simulink model "CF010A_GmTqArbn"  (R2013b)
settings: Solver=FixedStepDiscrete  SolverMode=SingleTasking  StartTime=0.0  StopTime=1  FixedStep=0.002  RelTol=1e-3
values from neighbouring files (symbols this model uses):
  ARCHGLBPRM_2MILLISEC_SEC_F32 = DataDict.Constant    [CF010A_GmTqArbn_DataDict.m]
  ESCTQCMDOVRLLIM_HWNWTMTR_F32 = DataDict.Constant    [CF010A_GmTqArbn_DataDict.m]
  FINALSLEWLWRLIM_HWNWTMTRPERSEC_F32 = DataDict.Constant    [CF010A_GmTqArbn_DataDict.m]
  GmTqArbnApaAssiScaEna = DataDict.Calibration    [CF010A_GmTqArbn_DataDict.m]
  GmTqArbnApaDampgScaEna = DataDict.Calibration    [CF010A_GmTqArbn_DataDict.m]
  GmTqArbnApaEnaRate = DataDict.Calibration    [CF010A_GmTqArbn_DataDict.m]
  GmTqArbnApaRtnScaEna = DataDict.Calibration    [CF010A_GmTqArbn_DataDict.m]
  GmTqArbnEscMaxTq = DataDict.Calibration    [CF010A_GmTqArbn_DataDict.m]
  GmTqArbnLkaOutpOvrlUpprLim = DataDict.Calibration    [CF010A_GmTqArbn_DataDict.m]
  GmTqArbnLkaSlewEna = DataDict.Calibration    [CF010A_GmTqArbn_DataDict.m]
  HWTQCMDOVRLLIM_HWNWTMTR_F32 = DataDict.Constant    [CF010A_GmTqArbn_DataDict.m]
  LKACMDHILIM_HWNWTMTR_F32 = DataDict.Constant    [CF010A_GmTqArbn_DataDict.m]
  LKAOUTPOVRLLIM_MOTNWTMTR_F32 = DataDict.Constant    [CF010A_GmTqArbn_DataDict.m]
  LKATQCMDOVRLLIM_HWNWTMTR_F32 = DataDict.Constant    [CF010A_GmTqArbn_DataDict.m]
  MOTTQCMDOVRLLIM_MOTNWTMTR_F32 = DataDict.Constant    [CF010A_GmTqArbn_DataDict.m]
  OUTPCMDHILIM_ULS_F32 = DataDict.Constant    [CF010A_GmTqArbn_DataDict.m]
  OUTPCMDLOWRLIM_ULS_F32 = DataDict.Constant    [CF010A_GmTqArbn_DataDict.m]
  POSNSERVOSMOOTHMINLWRLIM_ULSPERSEC_F32 = DataDict.Constant    [CF010A_GmTqArbn_DataDict.m]
  VELDPTTQOVRLMTRCOFFS_HWNWTMTRPERSEC_F32 = DataDict.Constant    [CF010A_GmTqArbn_DataDict.m]
  VELDPTTQOVRLMTRCTQPERVEHSPD_HWNWTMTRPERSECPERKPH_F32 = DataDict.Constant    [CF010A_GmTqArbn_DataDict.m]
undefined symbols (not defined in the file or in its folder): GmTqArbnEscSt1, GmTqArbnLkaSt1
libraries: NxtrLim x12, simulink x10, NexteerUtilities x8, FixdToFloat x4, NxtrAbslt x3, Fil x2, FloatToFixd x2, BilnrIntrpnMplX x1, NxtrSign x1
(part 4 of 5)

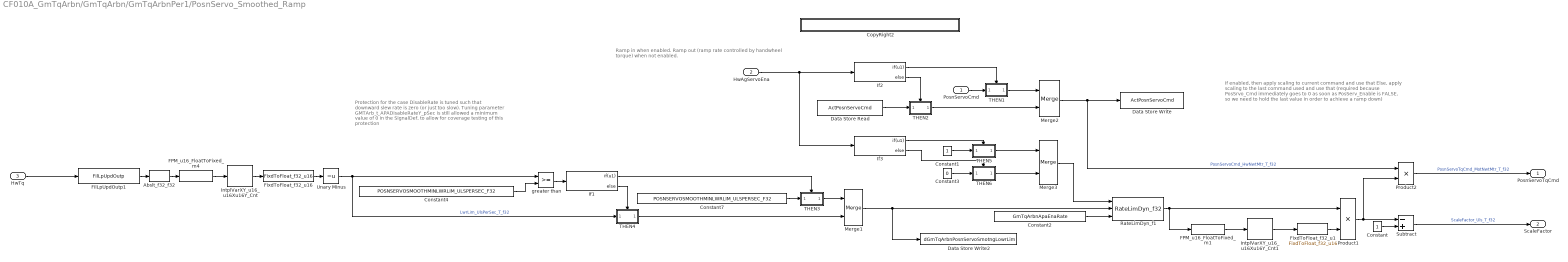
== system CF010A_GmTqArbn/GmTqArbn/GmTqArbnPer1/PosnServo_Smoothed_Ramp ==
  note: Protection for the case DisableRate is tuned such that
      | downward slew rate is zero (or just too slow).
      |
      | Tuning parameter GMTArb_t_APADisableRateY_pSec is still
      | allowed a minimum value of 0 in the SignalDef, to allow for
      | coverage testing of this protection
  note: Ramp in when enabled.
      | Ramp out (ramp rate controlled by handwheel torque) when not enabled.
  note: If enabled,
      |     then apply scaling to current command and use that
      | Else,
      |     apply scaling to the last command used and use that
      |
      |           (required because PosSrvo_Cmd immediately goes to 0 as soon
      |            as PosServ_Enable is FALSE, so we need to hold the last value
      |            in order to achieve a ramp down)
  PosnServoCmd : Inport  RequirementInfo="{'linktype_rmi_doors' '0000c6e3 (/E-STEER Core/SubSystem Specifications/Customer Functions - EA4/GM/CF010A GM Torque Arbitrator)' '#CF010A_83' 'true' 'REQ:  CF010A_83' '' } %GIDa_a589d5a5_5fe7_4259_9e30_a8e3d0a14d84"
  HwAgServoEna : Inport  RequirementInfo="{'linktype_rmi_doors' '0000c6e3 (/E-STEER Core/SubSystem Specifications/Customer Functions - EA4/GM/CF010A GM Torque Arbitrator)' '#CF010A_83' 'true' 'REQ:  CF010A_83' '' } %GIDa_3c39fabe_76d8_4d75_b934_ff4ece5048a2"  Port=2
  HwTq : Inport  RequirementInfo="{'linktype_rmi_doors' '0000c6e3 (/E-STEER Core/SubSystem Specifications/Customer Functions - EA4/GM/CF010A GM Torque Arbitrator)' '#CF010A_85' 'true' 'REQ:  CF010A_85' '' } %GIDa_14a06130_4ede_469d_aba7_55d801ee6fbb"  Port=3
  Abslt_f32_f32 : NxtrAbslt/Abslt_f32_f32  RequirementInfo="{'linktype_rmi_doors' '0000c6e3 (/E-STEER Core/SubSystem Specifications/Customer Functions - EA4/GM/CF010A GM Torque Arbitrator)' '#CF010A_85' 'true' 'REQ:  CF010A_85' '' } %GIDa_1d732af2_bae1_4918_9fbb_75956b3de41a"  SFunctionSpec=single y1 = Abslt_f32_f32(single u1)
      settings: AttributesFormatString=%<Name>
  Constant : Constant  RequirementInfo="{'linktype_rmi_doors' '0000c6e3 (/E-STEER Core/SubSystem Specifications/Customer Functions - EA4/GM/CF010A GM Torque Arbitrator)' '#CF010A_87' 'true' 'REQ:  CF010A_87' '' } %GIDa_6652223e_5f9e_4f22_b2f7_82ef07e16371"  OutDataTypeStr=single
  Constant1 : Constant  RequirementInfo="{'linktype_rmi_doors' '0000c6e3 (/E-STEER Core/SubSystem Specifications/Customer Functions - EA4/GM/CF010A GM Torque Arbitrator)' '#CF010A_83' 'true' 'REQ:  CF010A_83' '' } %GIDa_8a974f93_c71b_4ff7_97b8_e3459b4cb0d6"  OutDataTypeStr=single
  Constant2 : Constant  RequirementInfo="{'linktype_rmi_doors' '0000c6e3 (/E-STEER Core/SubSystem Specifications/Customer Functions - EA4/GM/CF010A GM Torque Arbitrator)' '#CF010A_84' 'true' 'REQ:  CF010A_84' '' } %GIDa_7ed8c832_ce99_4127_9a80_eb8922502510"  Value=GmTqArbnApaEnaRate
  Constant3 : Constant  RequirementInfo="{'linktype_rmi_doors' '0000c6e3 (/E-STEER Core/SubSystem Specifications/Customer Functions - EA4/GM/CF010A GM Torque Arbitrator)' '#CF010A_83' 'true' 'REQ:  CF010A_83' '' } %GIDa_389fbbe5_3959_44b2_9e53_45f6397d449f"  Value=0  OutDataTypeStr=single
  Constant4 : Constant  RequirementInfo={} %GIDa_c73b5d52_2f1d_4595_892c_5347f865968c  Value=POSNSERVOSMOOTHMINLWRLIM_ULSPERSEC_F32
  Constant7 : Constant  RequirementInfo={} %GIDa_8f1476cf_19b2_4cf1_8322_e9f8d22341c9  Value=POSNSERVOSMOOTHMINLWRLIM_ULSPERSEC_F32
  CopyRight2 : Subsystem  Description=|  mask(Copyright Information){none=on}
      | Copyright info block.                                               
      |                                                                     
      | Place copyright information at the top of every subsystem in design.
      mask prompts: none "No parameters"
      mask help: Place copyright information at the top of every subsystem in design.
      mask Display:
      | NxtrConf = 'Nexteer Confidential';
      | 
      | sys = bdroot; %handle for the current model ("system")
      | first = get_param(sys,'Created');
      | first = first(end-3:end);  %year is last four digits
      | 
      | last = get_param(sys,'LastModifiedDate');
      | if isempty(last)
      |     last = datestr(now,'yyyy');
      | else
      |     last = last(end-3:end);
      | end
      | 
      | if strcmp(first,last)
      |     fprintf('%s -- Copyright %s Nexteer',NxtrConf,first)
      | else
      |     fprintf('%s -- %s%s- %s Nexteer',NxtrConf,char(169),first,last)
      | end
  Data Store Read : DataStoreRead  RequirementInfo="{'linktype_rmi_doors' '0000c6e3 (/E-STEER Core/SubSystem Specifications/Customer Functions - EA4/GM/CF010A GM Torque Arbitrator)' '#CF010A_83' 'true' 'REQ:  CF010A_83' '' } %GIDa_2b8eed64_a4c6_49b0_96b2_799e9470223f"  DataStoreName=ActPosnServoCmd
  Data Store Write : DataStoreWrite  RequirementInfo="{'linktype_rmi_doors' '0000c6e3 (/E-STEER Core/SubSystem Specifications/Customer Functions - EA4/GM/CF010A GM Torque Arbitrator)' '#CF010A_83' 'true' 'REQ:  CF010A_83' '' } %GIDa_49e27e17_eee5_40eb_b093_ed4163babafd"  DataStoreName=ActPosnServoCmd
  Data Store Write2 : DataStoreWrite  DataStoreName=dGmTqArbnPosnServoSmotngLowrLim
  FPM_u16_FloatToFixed_m1 : NexteerUtilities/Fixed Point Math Conversions/FPM_u16_FloatToFixed_m  RequirementInfo="{'linktype_rmi_doors' '0000c6e3 (/E-STEER Core/SubSystem Specifications/Customer Functions - EA4/GM/CF010A GM Torque Arbitrator)' '#CF010A_87' 'true' 'REQ:  CF010A_87' '' } %GIDa_42565968_b0f1_480f_9ffe_acf6ef03b720"  SFunctionSpec=uint16 y1 = FPM_u16_FloatToFixed_m(single u1, single p1)  Param1=15
      settings: AttributesFormatString=u16_FloatToFixed
  FPM_u16_FloatToFixed_m4 : NexteerUtilities/Fixed Point Math Conversions/FPM_u16_FloatToFixed_m  RequirementInfo="{'linktype_rmi_doors' '0000c6e3 (/E-STEER Core/SubSystem Specifications/Customer Functions - EA4/GM/CF010A GM Torque Arbitrator)' '#CF010A_85' 'true' 'REQ:  CF010A_85' '' } %GIDa_11a7f01b_449d_4110_953e_6440d8c88ec2"  SFunctionSpec=uint16 y1 = FPM_u16_FloatToFixed_m(single u1, single p1)  Param1=12
      settings: AttributesFormatString=u16_FloatToFixed
  FilLpUpdOutp1 : Fil/FilLpUpdOutp  RequirementInfo="{'linktype_rmi_doors' '0000c6e3 (/E-STEER Core/SubSystem Specifications/Customer Functions - EA4/GM/CF010A GM Torque Arbitrator)' '#CF010A_85' 'true' 'REQ:  CF010A_85' '' } %GIDa_6001f4fc_91a0_455a_8ef8_6b05b3874b38"  StVar=ApaSmotngHwTqLpFil
      settings: AttributesFormatString=StVar: %<StVar>
  FixdToFloat_f32_u1 : FixdToFloat/FixdToFloat_f32_u16  RequirementInfo="{'linktype_rmi_doors' '0000c6e3 (/E-STEER Core/SubSystem Specifications/Customer Functions - EA4/GM/CF010A GM Torque Arbitrator)' '#CF010A_87' 'true' 'REQ:  CF010A_87' '' } %GIDa_01cc822d_a521_45f2_8614_de07a41cf4e7"  Param1=15
  FixdToFloat_f32_u16 : FixdToFloat/FixdToFloat_f32_u16  RequirementInfo="{'linktype_rmi_doors' '0000c6e3 (/E-STEER Core/SubSystem Specifications/Customer Functions - EA4/GM/CF010A GM Torque Arbitrator)' '#CF010A_85' 'true' 'REQ:  CF010A_85' '' } %GIDa_d247bf31_8ee9_41f8_b2ef_9ed7cd29173a"  Param1=9
  If1 : If  RequirementInfo={} %GIDa_446387ce_f822_476d_a5ec_ea0813341457  IfExpression=u1
  If2 : If  RequirementInfo="{'linktype_rmi_doors' '0000c6e3 (/E-STEER Core/SubSystem Specifications/Customer Functions - EA4/GM/CF010A GM Torque Arbitrator)' '#CF010A_83' 'true' 'REQ:  CF010A_83' '' } %GIDa_caed38e4_3d6b_4104_9897_516a2005e0ea"  IfExpression=u1
  If3 : If  RequirementInfo="{'linktype_rmi_doors' '0000c6e3 (/E-STEER Core/SubSystem Specifications/Customer Functions - EA4/GM/CF010A GM Torque Arbitrator)' '#CF010A_83' 'true' 'REQ:  CF010A_83' '' } %GIDa_cb067983_f98e_478f_9a9b_9a4768f0638b"  IfExpression=u1
  IntplVarXY_u16_u16Xu16Y_Cnt : NexteerUtilities/Interpolation/IntplVarXY_u16_u16Xu16Y_Cnt  RequirementInfo="{'linktype_rmi_doors' '0000c6e3 (/E-STEER Core/SubSystem Specifications/Customer Functions - EA4/GM/CF010A GM Torque Arbitrator)' '#CF010A_85' 'true' 'REQ:  CF010A_85' '' } %GIDa_c034638a_826b_4a44_a2db_ef50f5019c4a"  Param1=GmTqArbnApaDiRateX  Param2=GmTqArbnApaDiRateY
      settings: AttributesFormatString=IntplVarXY (uX, uY)
  IntplVarXY_u16_u16Xu16Y_Cnt1 : NexteerUtilities/Interpolation/IntplVarXY_u16_u16Xu16Y_Cnt  RequirementInfo="{'linktype_rmi_doors' '0000c6e3 (/E-STEER Core/SubSystem Specifications/Customer Functions - EA4/GM/CF010A GM Torque Arbitrator)' '#CF010A_87' 'true' 'REQ:  CF010A_87' '' ; 'linktype_rmi_doors' '0000c6e3 (/E-STEER Core/SubSystem Specifications/Customer Functions - EA4/GM/CF010A GM Torque Arbitrator)' '#CF010A_86' 'true' 'REQ:  CF010A_86' '' } %GIDa_d2f04c6c_cd0d_4f5b_a0ee_624f7a3ac7bb"  Param1=GmTqArbnApaSmotngX  Param2=GmTqArbnApaSmotngY
      settings: AttributesFormatString=IntplVarXY (uX, uY)
  Merge1 : Merge  RequirementInfo={} %GIDa_c6bad38d_cfbe_4ba5_8efa_e31f6e6c40e4
  Merge2 : Merge  RequirementInfo="{'linktype_rmi_doors' '0000c6e3 (/E-STEER Core/SubSystem Specifications/Customer Functions - EA4/GM/CF010A GM Torque Arbitrator)' '#CF010A_83' 'true' 'REQ:  CF010A_83' '' } %GIDa_315cc2c9_a434_4900_996a_ec94b76d111f"
  Merge3 : Merge  RequirementInfo="{'linktype_rmi_doors' '0000c6e3 (/E-STEER Core/SubSystem Specifications/Customer Functions - EA4/GM/CF010A GM Torque Arbitrator)' '#CF010A_83' 'true' 'REQ:  CF010A_83' '' } %GIDa_22e32ead_0ffe_4af6_9c30_1dceeecbc313"
  Product1 : Product  RequirementInfo="{'linktype_rmi_doors' '0000c6e3 (/E-STEER Core/SubSystem Specifications/Customer Functions - EA4/GM/CF010A GM Torque Arbitrator)' '#CF010A_87' 'true' 'REQ:  CF010A_87' '' } %GIDa_d490a3f1_7ea3_496c_9645_bccc177abc5b"  OutDataTypeStr=single  RndMeth=Zero
  Product2 : Product  RequirementInfo="{'linktype_rmi_doors' '0000c6e3 (/E-STEER Core/SubSystem Specifications/Customer Functions - EA4/GM/CF010A GM Torque Arbitrator)' '#CF010A_86' 'true' 'REQ:  CF010A_86' '' } %GIDa_1ff153b9_865b_4418_aa1c_8853e303e2f0"  OutDataTypeStr=single  RndMeth=Zero
  RateLimDyn_f1 : NxtrLim/RateLimDyn_f32  RequirementInfo="{'linktype_rmi_doors' '0000c6e3 (/E-STEER Core/SubSystem Specifications/Customer Functions - EA4/GM/CF010A GM Torque Arbitrator)' '#CF010A_84' 'true' 'REQ:  CF010A_84' '' } %GIDa_4a1a811f_29b7_4717_8310_006cae323995"  StVar=PosnServoSmotngEnaRateLim  Ts=ARCHGLBPRM_2MILLISEC_SEC_F32
      settings: AttributesFormatString=StVar: %<StVar>
  Subtract : Sum  RequirementInfo="{'linktype_rmi_doors' '0000c6e3 (/E-STEER Core/SubSystem Specifications/Customer Functions - EA4/GM/CF010A GM Torque Arbitrator)' '#CF010A_87' 'true' 'REQ:  CF010A_87' '' } %GIDa_3c2bba99_87d7_4ba6_923a_93c919a35035"  Inputs=-+
  THEN1 : Subsystem  RequirementInfo="{'linktype_rmi_doors' '0000c6e3 (/E-STEER Core/SubSystem Specifications/Customer Functions - EA4/GM/CF010A GM Torque Arbitrator)' '#CF010A_83' 'true' 'REQ:  CF010A_83' '' } %GIDa_80c3f70f_6981_41a7_879d_713cfb9f3918"  TreatAsAtomicUnit=on  mask(pass thru, version Nov 30, 2012){nIn=1}
      mask prompts: nIn "Number of input signals"
      mask help:
      | This block passes its input straight through without modification.
      |
      | Enter the number of signals to pass through (integer 1 to 5).
      mask Callback nIn:
      | thisBlock = gcb;
      | a = get_param(thisBlock,'MaskValues');
      | b = cell2mat(a);
      | c = str2num(b);
      | 
      | if c<1 c=1; end
      | if c>5 c=5; end
      | 
      | for idx=1:c
      |     sIdx = num2str(idx);
      |     oldblock = [thisBlock '/In' sIdx];
      |     if strcmp(get_param(oldblock,'BlockType'),'Ground')
      |          newblock = 'built-in/Inport';
      |         pos = get_param(oldblock,'Position');
      |         orient = get_param(oldblock,'Orientation');
      |         delete_block(oldblock);
      |         add_block(newblock,oldblock,'Position',pos, 'Orientation',orient);
      |     end
      | 
      |     oldblock = [thisBlock '/Out' sIdx];
      |     if strcmp(get_param(oldblock,'BlockType'),'Terminator')
      |         newblock = 'built-in/Outport';
      |         pos = get_param(oldblock,'Position');
      |         orient = get_param(oldblock,'Orientation');
      |         delete_block(oldblock);
      |         add_block(newblock,oldblock,'Position',pos, 'Orientation',orient);
      |     end
      | end
      | 
      | for idx=c+1:5
      |     sIdx = num2str(idx);
      |     oldblock = [thisBlock '/In' sIdx];
      |     if strcmp(get_param(oldblock,'BlockType'),'Inport')
      |         newblock = 'built-in/Ground';
      |         pos = get_param(oldblock,'Position');
      |         orient = get_param(oldblock,'Orientation');
      |         delete_block(oldblock);
      |         add_block(newblock,oldblock,'Position',pos, 'Orientation',orient);
      |     end
      | 
      |     oldblock = [thisBlock '/Out' sIdx];
      |     if strcmp(get_param(oldblock,'BlockType'),'Outport')
      |         newblock = 'built-in/Terminator';
      |         pos = get_param(oldblock,'Position');
      |         orient = get_param(oldblock,'Orientation');
      |         delete_block(oldblock);
      |         add_block(newblock,oldblock,'Position',pos, 'Orientation',orient);
      |     end
      | end
      | 
      | 
      | 
      | clear thisBlock oldblock newblock orient pos a b c idx sIdx ;
      mask Display: fprintf('pass\nthru')
  THEN2 : Subsystem  RequirementInfo="{'linktype_rmi_doors' '0000c6e3 (/E-STEER Core/SubSystem Specifications/Customer Functions - EA4/GM/CF010A GM Torque Arbitrator)' '#CF010A_83' 'true' 'REQ:  CF010A_83' '' } %GIDa_f9d28e7a_0d49_44fe_8c5c_4cae6e915892"  TreatAsAtomicUnit=on  mask(pass thru, version Nov 30, 2012){nIn=1}
      mask prompts: nIn "Number of input signals"
      mask help:
      | This block passes its input straight through without modification.
      |
      | Enter the number of signals to pass through (integer 1 to 5).
      mask Callback nIn:
      | thisBlock = gcb;
      | a = get_param(thisBlock,'MaskValues');
      | b = cell2mat(a);
      | c = str2num(b);
      | 
      | if c<1 c=1; end
      | if c>5 c=5; end
      | 
      | for idx=1:c
      |     sIdx = num2str(idx);
      |     oldblock = [thisBlock '/In' sIdx];
      |     if strcmp(get_param(oldblock,'BlockType'),'Ground')
      |          newblock = 'built-in/Inport';
      |         pos = get_param(oldblock,'Position');
      |         orient = get_param(oldblock,'Orientation');
      |         delete_block(oldblock);
      |         add_block(newblock,oldblock,'Position',pos, 'Orientation',orient);
      |     end
      | 
      |     oldblock = [thisBlock '/Out' sIdx];
      |     if strcmp(get_param(oldblock,'BlockType'),'Terminator')
      |         newblock = 'built-in/Outport';
      |         pos = get_param(oldblock,'Position');
      |         orient = get_param(oldblock,'Orientation');
      |         delete_block(oldblock);
      |         add_block(newblock,oldblock,'Position',pos, 'Orientation',orient);
      |     end
      | end
      | 
      | for idx=c+1:5
      |     sIdx = num2str(idx);
      |     oldblock = [thisBlock '/In' sIdx];
      |     if strcmp(get_param(oldblock,'BlockType'),'Inport')
      |         newblock = 'built-in/Ground';
      |         pos = get_param(oldblock,'Position');
      |         orient = get_param(oldblock,'Orientation');
      |         delete_block(oldblock);
      |         add_block(newblock,oldblock,'Position',pos, 'Orientation',orient);
      |     end
      | 
      |     oldblock = [thisBlock '/Out' sIdx];
      |     if strcmp(get_param(oldblock,'BlockType'),'Outport')
      |         newblock = 'built-in/Terminator';
      |         pos = get_param(oldblock,'Position');
      |         orient = get_param(oldblock,'Orientation');
      |         delete_block(oldblock);
      |         add_block(newblock,oldblock,'Position',pos, 'Orientation',orient);
      |     end
      | end
      | 
      | 
      | 
      | clear thisBlock oldblock newblock orient pos a b c idx sIdx ;
      mask Display: fprintf('pass\nthru')
  THEN3 : Subsystem  RequirementInfo={} %GIDa_d57778e5_423b_47fa_b317_4be07015d79c  TreatAsAtomicUnit=on  mask(pass thru, version Nov 30, 2012){nIn=1}
      mask prompts: nIn "Number of input signals"
      mask help:
      | This block passes its input straight through without modification.
      |
      | Enter the number of signals to pass through (integer 1 to 5).
      mask Callback nIn:
      | thisBlock = gcb;
      | a = get_param(thisBlock,'MaskValues');
      | b = cell2mat(a);
      | c = str2num(b);
      | 
      | if c<1 c=1; end
      | if c>5 c=5; end
      | 
      | for idx=1:c
      |     sIdx = num2str(idx);
      |     oldblock = [thisBlock '/In' sIdx];
      |     if strcmp(get_param(oldblock,'BlockType'),'Ground')
      |          newblock = 'built-in/Inport';
      |         pos = get_param(oldblock,'Position');
      |         orient = get_param(oldblock,'Orientation');
      |         delete_block(oldblock);
      |         add_block(newblock,oldblock,'Position',pos, 'Orientation',orient);
      |     end
      | 
      |     oldblock = [thisBlock '/Out' sIdx];
      |     if strcmp(get_param(oldblock,'BlockType'),'Terminator')
      |         newblock = 'built-in/Outport';
      |         pos = get_param(oldblock,'Position');
      |         orient = get_param(oldblock,'Orientation');
      |         delete_block(oldblock);
      |         add_block(newblock,oldblock,'Position',pos, 'Orientation',orient);
      |     end
      | end
      | 
      | for idx=c+1:5
      |     sIdx = num2str(idx);
      |     oldblock = [thisBlock '/In' sIdx];
      |     if strcmp(get_param(oldblock,'BlockType'),'Inport')
      |         newblock = 'built-in/Ground';
      |         pos = get_param(oldblock,'Position');
      |         orient = get_param(oldblock,'Orientation');
      |         delete_block(oldblock);
      |         add_block(newblock,oldblock,'Position',pos, 'Orientation',orient);
      |     end
      | 
      |     oldblock = [thisBlock '/Out' sIdx];
      |     if strcmp(get_param(oldblock,'BlockType'),'Outport')
      |         newblock = 'built-in/Terminator';
      |         pos = get_param(oldblock,'Position');
      |         orient = get_param(oldblock,'Orientation');
      |         delete_block(oldblock);
      |         add_block(newblock,oldblock,'Position',pos, 'Orientation',orient);
      |     end
      | end
      | 
      | 
      | 
      | clear thisBlock oldblock newblock orient pos a b c idx sIdx ;
      mask Display: fprintf('pass\nthru')
  THEN4 : Subsystem  RequirementInfo={} %GIDa_3f4dfbb6_d451_4e7e_94d4_863f405e7908  TreatAsAtomicUnit=on  mask(pass thru, version Nov 30, 2012){nIn=1}
      mask prompts: nIn "Number of input signals"
      mask help:
      | This block passes its input straight through without modification.
      |
      | Enter the number of signals to pass through (integer 1 to 5).
      mask Callback nIn:
      | thisBlock = gcb;
      | a = get_param(thisBlock,'MaskValues');
      | b = cell2mat(a);
      | c = str2num(b);
      | 
      | if c<1 c=1; end
      | if c>5 c=5; end
      | 
      | for idx=1:c
      |     sIdx = num2str(idx);
      |     oldblock = [thisBlock '/In' sIdx];
      |     if strcmp(get_param(oldblock,'BlockType'),'Ground')
      |          newblock = 'built-in/Inport';
      |         pos = get_param(oldblock,'Position');
      |         orient = get_param(oldblock,'Orientation');
      |         delete_block(oldblock);
      |         add_block(newblock,oldblock,'Position',pos, 'Orientation',orient);
      |     end
      | 
      |     oldblock = [thisBlock '/Out' sIdx];
      |     if strcmp(get_param(oldblock,'BlockType'),'Terminator')
      |         newblock = 'built-in/Outport';
      |         pos = get_param(oldblock,'Position');
      |         orient = get_param(oldblock,'Orientation');
      |         delete_block(oldblock);
      |         add_block(newblock,oldblock,'Position',pos, 'Orientation',orient);
      |     end
      | end
      | 
      | for idx=c+1:5
      |     sIdx = num2str(idx);
      |     oldblock = [thisBlock '/In' sIdx];
      |     if strcmp(get_param(oldblock,'BlockType'),'Inport')
      |         newblock = 'built-in/Ground';
      |         pos = get_param(oldblock,'Position');
      |         orient = get_param(oldblock,'Orientation');
      |         delete_block(oldblock);
      |         add_block(newblock,oldblock,'Position',pos, 'Orientation',orient);
      |     end
      | 
      |     oldblock = [thisBlock '/Out' sIdx];
      |     if strcmp(get_param(oldblock,'BlockType'),'Outport')
      |         newblock = 'built-in/Terminator';
      |         pos = get_param(oldblock,'Position');
      |         orient = get_param(oldblock,'Orientation');
      |         delete_block(oldblock);
      |         add_block(newblock,oldblock,'Position',pos, 'Orientation',orient);
      |     end
      | end
      | 
      | 
      | 
      | clear thisBlock oldblock newblock orient pos a b c idx sIdx ;
      mask Display: fprintf('pass\nthru')
  THEN5 : Subsystem  RequirementInfo="{'linktype_rmi_doors' '0000c6e3 (/E-STEER Core/SubSystem Specifications/Customer Functions - EA4/GM/CF010A GM Torque Arbitrator)' '#CF010A_83' 'true' 'REQ:  CF010A_83' '' } %GIDa_1fd1b70b_60eb_42bd_bdff_5612c0d9123a"  TreatAsAtomicUnit=on  mask(pass thru, version Nov 30, 2012){nIn=1}
      mask prompts: nIn "Number of input signals"
      mask help:
      | This block passes its input straight through without modification.
      |
      | Enter the number of signals to pass through (integer 1 to 5).
      mask Callback nIn:
      | thisBlock = gcb;
      | a = get_param(thisBlock,'MaskValues');
      | b = cell2mat(a);
      | c = str2num(b);
      | 
      | if c<1 c=1; end
      | if c>5 c=5; end
      | 
      | for idx=1:c
      |     sIdx = num2str(idx);
      |     oldblock = [thisBlock '/In' sIdx];
      |     if strcmp(get_param(oldblock,'BlockType'),'Ground')
      |          newblock = 'built-in/Inport';
      |         pos = get_param(oldblock,'Position');
      |         orient = get_param(oldblock,'Orientation');
      |         delete_block(oldblock);
      |         add_block(newblock,oldblock,'Position',pos, 'Orientation',orient);
      |     end
      | 
      |     oldblock = [thisBlock '/Out' sIdx];
      |     if strcmp(get_param(oldblock,'BlockType'),'Terminator')
      |         newblock = 'built-in/Outport';
      |         pos = get_param(oldblock,'Position');
      |         orient = get_param(oldblock,'Orientation');
      |         delete_block(oldblock);
      |         add_block(newblock,oldblock,'Position',pos, 'Orientation',orient);
      |     end
      | end
      | 
      | for idx=c+1:5
      |     sIdx = num2str(idx);
      |     oldblock = [thisBlock '/In' sIdx];
      |     if strcmp(get_param(oldblock,'BlockType'),'Inport')
      |         newblock = 'built-in/Ground';
      |         pos = get_param(oldblock,'Position');
      |         orient = get_param(oldblock,'Orientation');
      |         delete_block(oldblock);
      |         add_block(newblock,oldblock,'Position',pos, 'Orientation',orient);
      |     end
      | 
      |     oldblock = [thisBlock '/Out' sIdx];
      |     if strcmp(get_param(oldblock,'BlockType'),'Outport')
      |         newblock = 'built-in/Terminator';
      |         pos = get_param(oldblock,'Position');
      |         orient = get_param(oldblock,'Orientation');
      |         delete_block(oldblock);
      |         add_block(newblock,oldblock,'Position',pos, 'Orientation',orient);
      |     end
      | end
      | 
      | 
      | 
      | clear thisBlock oldblock newblock orient pos a b c idx sIdx ;
      mask Display: fprintf('pass\nthru')
  THEN6 : Subsystem  RequirementInfo="{'linktype_rmi_doors' '0000c6e3 (/E-STEER Core/SubSystem Specifications/Customer Functions - EA4/GM/CF010A GM Torque Arbitrator)' '#CF010A_83' 'true' 'REQ:  CF010A_83' '' } %GIDa_adb91255_bd60_4dba_91f8_f7c9d20f79bd"  TreatAsAtomicUnit=on  mask(pass thru, version Nov 30, 2012){nIn=1}
      mask prompts: nIn "Number of input signals"
      mask help:
      | This block passes its input straight through without modification.
      |
      | Enter the number of signals to pass through (integer 1 to 5).
      mask Callback nIn:
      | thisBlock = gcb;
      | a = get_param(thisBlock,'MaskValues');
      | b = cell2mat(a);
      | c = str2num(b);
      | 
      | if c<1 c=1; end
      | if c>5 c=5; end
      | 
      | for idx=1:c
      |     sIdx = num2str(idx);
      |     oldblock = [thisBlock '/In' sIdx];
      |     if strcmp(get_param(oldblock,'BlockType'),'Ground')
      |          newblock = 'built-in/Inport';
      |         pos = get_param(oldblock,'Position');
      |         orient = get_param(oldblock,'Orientation');
      |         delete_block(oldblock);
      |         add_block(newblock,oldblock,'Position',pos, 'Orientation',orient);
      |     end
      | 
      |     oldblock = [thisBlock '/Out' sIdx];
      |     if strcmp(get_param(oldblock,'BlockType'),'Terminator')
      |         newblock = 'built-in/Outport';
      |         pos = get_param(oldblock,'Position');
      |         orient = get_param(oldblock,'Orientation');
      |         delete_block(oldblock);
      |         add_block(newblock,oldblock,'Position',pos, 'Orientation',orient);
      |     end
      | end
      | 
      | for idx=c+1:5
      |     sIdx = num2str(idx);
      |     oldblock = [thisBlock '/In' sIdx];
      |     if strcmp(get_param(oldblock,'BlockType'),'Inport')
      |         newblock = 'built-in/Ground';
      |         pos = get_param(oldblock,'Position');
      |         orient = get_param(oldblock,'Orientation');
      |         delete_block(oldblock);
      |         add_block(newblock,oldblock,'Position',pos, 'Orientation',orient);
      |     end
      | 
      |     oldblock = [thisBlock '/Out' sIdx];
      |     if strcmp(get_param(oldblock,'BlockType'),'Outport')
      |         newblock = 'built-in/Terminator';
      |         pos = get_param(oldblock,'Position');
      |         orient = get_param(oldblock,'Orientation');
      |         delete_block(oldblock);
      |         add_block(newblock,oldblock,'Position',pos, 'Orientation',orient);
      |     end
      | end
      | 
      | 
      | 
      | clear thisBlock oldblock newblock orient pos a b c idx sIdx ;
      mask Display: fprintf('pass\nthru')
  Unary Minus : UnaryMinus  RequirementInfo="{'linktype_rmi_doors' '0000c6e3 (/E-STEER Core/SubSystem Specifications/Customer Functions - EA4/GM/CF010A GM Torque Arbitrator)' '#CF010A_85' 'true' 'REQ:  CF010A_85' '' } %GIDa_b5598d6e_8cf5_4f78_a293_b87017c84204"
  greater than : RelationalOperator  RequirementInfo={} %GIDa_87b77e6d_940b_4ccf_b202_250e23c15458  OutDataTypeStr=boolean
  PosnServoTqCmd : Outport  RequirementInfo="{'linktype_rmi_doors' '0000c6e3 (/E-STEER Core/SubSystem Specifications/Customer Functions - EA4/GM/CF010A GM Torque Arbitrator)' '#CF010A_86' 'true' 'REQ:  CF010A_86' '' } %GIDa_a4b38a79_013d_43b6_9898_556ebefc35fa"
  ScaleFactor : Outport  RequirementInfo="{'linktype_rmi_doors' '0000c6e3 (/E-STEER Core/SubSystem Specifications/Customer Functions - EA4/GM/CF010A GM Torque Arbitrator)' '#CF010A_87' 'true' 'REQ:  CF010A_87' '' } %GIDa_643bb415_ec35_4a05_a47c_19160a6da6bf"  Port=2
  wires:
  Merge2/1 -> Product2/1, Data Store Write/1  "PosnServoCmd_HwNwtMtr_T_f32"
  Product1/1 -> Subtract/1, Product2/2
  Constant/1 -> Subtract/2
  Product2/1 -> PosnServoTqCmd/1  "PosnServoTqCmd_MotNwtMtr_T_f32"
  Subtract/1 -> ScaleFactor/1  "ScaleFactor_Uls_T_f32"
  RateLimDyn_f1/1 -> Product1/1, FPM_u16_FloatToFixed_m1/1
  Constant2/1 -> RateLimDyn_f1/3
  Merge3/1 -> RateLimDyn_f1/1
  FixdToFloat_f32_u16/1 -> Unary Minus/1
  FixdToFloat_f32_u1/1 -> Product1/2
  Merge1/1 -> Data Store Write2/1, RateLimDyn_f1/2
  IntplVarXY_u16_u16Xu16Y_Cnt/1 -> FixdToFloat_f32_u16/1
  FPM_u16_FloatToFixed_m4/1 -> IntplVarXY_u16_u16Xu16Y_Cnt/1
  Abslt_f32_f32/1 -> FPM_u16_FloatToFixed_m4/1
  FilLpUpdOutp1/1 -> Abslt_f32_f32/1
  Constant4/1 -> greater than/2
  THEN3/1(Out1) -> Merge1/1
  Constant7/1 -> THEN3/1(In1)
  If1/1 -> THEN3/Action
  Unary Minus/1 -> greater than/1, THEN4/1(In1)  "LwrLim_UlsPerSec_T_f32"
  If1/2 -> THEN4/Action
  THEN4/1(Out1) -> Merge1/2
  greater than/1 -> If1/1
  IntplVarXY_u16_u16Xu16Y_Cnt1/1 -> FixdToFloat_f32_u1/1
  FPM_u16_FloatToFixed_m1/1 -> IntplVarXY_u16_u16Xu16Y_Cnt1/1
  Data Store Read/1 -> THEN2/1(In1)
  THEN1/1(Out1) -> Merge2/1
  If2/1 -> THEN1/Action
  If2/2 -> THEN2/Action
  THEN2/1(Out1) -> Merge2/2
  If3/1 -> THEN5/Action
  If3/2 -> THEN6/Action
  Constant3/1 -> THEN6/1(In1)
  THEN5/1(Out1) -> Merge3/1
  THEN6/1(Out1) -> Merge3/2
  HwAgServoEna/1 -> If3/1, If2/1
  PosnServoCmd/1 -> THEN1/1(In1)
  Constant1/1 -> THEN5/1(In1)
  HwTq/1 -> FilLpUpdOutp1/1

== system CF010A_GmTqArbn/GmTqArbn/GmTqArbnPer1/Pull Compensation Learning Trigger ==
  ESCActv : Inport
  LkaSt : Inport  Port=2
  CopyRight2 : Subsystem  Description=|  mask(Copyright Information){none=on}
      | Copyright info block.                                               
      |                                                                     
      | Place copyright information at the top of every subsystem in design.
      mask prompts: none "No parameters"
      mask help: Place copyright information at the top of every subsystem in design.
      mask Display:
      | NxtrConf = 'Nexteer Confidential';
      | 
      | sys = bdroot; %handle for the current model ("system")
      | first = get_param(sys,'Created');
      | first = first(end-3:end);  %year is last four digits
      | 
      | last = get_param(sys,'LastModifiedDate');
      | if isempty(last)
      |     last = datestr(now,'yyyy');
      | else
      |     last = last(end-3:end);
      | end
      | 
      | if strcmp(first,last)
      |     fprintf('%s -- Copyright %s Nexteer',NxtrConf,first)
      | else
      |     fprintf('%s -- %s%s- %s Nexteer',NxtrConf,char(169),first,last)
      | end
  Enumerated Constant : simulink/Sources/Enumerated Constant  OutDataTypeStr=Enum: GmTqArbnLkaSt1  Value=GmTqArbnLkaSt1.GMTQARBNLKAST_ACTV  SampleTime=inf
  Enumerated Constant1 : simulink/Sources/Enumerated Constant  OutDataTypeStr=Enum: GmTqArbnLkaSt1  Value=GmTqArbnLkaSt1.GMTQARBNLKAST_TMPLIMD  SampleTime=inf
  Logical Operator : Logic  Operator=OR  AllPortsSameDT=off  OutDataTypeStr=boolean
  Logical Operator1 : Logic  Operator=OR  AllPortsSameDT=off  OutDataTypeStr=boolean
  Relational Operator2 : RelationalOperator  Operator===  OutDataTypeStr=boolean
  Relational Operator3 : RelationalOperator  Operator===  OutDataTypeStr=boolean
  PullCmpCustLrngDi : Outport
  wires:
  Logical Operator1/1 -> Logical Operator/2
  LkaSt/1 -> Relational Operator2/1, Relational Operator3/1
  Relational Operator2/1 -> Logical Operator1/1
  ESCActv/1 -> Logical Operator/1
  Logical Operator/1 -> PullCmpCustLrngDi/1
  Relational Operator3/1 -> Logical Operator1/2
  Enumerated Constant/1 -> Relational Operator2/2
  Enumerated Constant1/1 -> Relational Operator3/2
